simulink model "Lab1_Part1"  (R2022b)
settings: Solver=VariableStepAuto  StartTime=0.0  StopTime=20.0  RelTol=1e-3
settings Model: Creator=Sahaj Singh  LastModifiedBy=Sahaj Singh

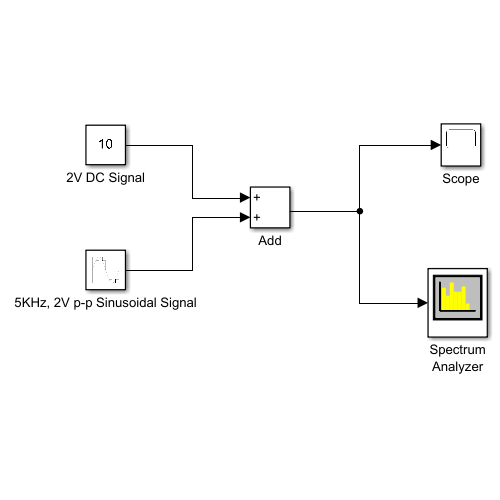
[thumbnail: Simulink's stored preview of the top-level diagram]
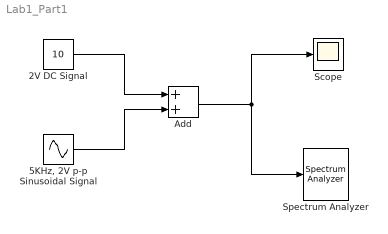
== system Lab1_Part1 ==
  2V DC Signal : Constant  Value=10
  "5KHz, 2V p-p Sinusoidal Signal" : Sin  Amplitude=2  Frequency=62831.853  SampleTime=1/5000
  Add : Sum
  Scope : Scope
  Spectrum Analyzer : SpectrumAnalyzer
  wires:
  2V DC Signal/1 -> Add/1
  "5KHz, 2V p-p Sinusoidal Signal"/1 -> Add/2
  Add/1 -> Scope/1, Spectrum Analyzer/1
